simulink model "VVI"  (R2022b)
settings: Solver=FixedStepAuto  StartTime=0.0  StopTime=10.0  FixedStep=1e-3  RelTol=1e-3  EnableMultiTasking=on
undefined symbols (not defined in the file): A0, D1, D10, D12, D2, D5, D9, PTA2, PTB2, PTB9, PTC17, PTC4, PTD0, PTD3
libraries: frdmk64flib x7
settings Model: ExtModeTrigDuration=5  Creator=peter  LastModifiedBy=Dhilan
settings OptimizationCC: EnhancedBackFolding=on  PassReuseOutputArgsAs=Individual arguments  ZeroExternalMemoryAtStartup=off  ZeroInternalMemoryAtStartup=off  MaxStackSize=64  OptimizeBlockOrder=speed  DifferentSizesBufferReuse=on  OptimizationCustomize=off  EfficientTunableParamExpr=on
settings DebuggingCC: ParameterTunabilityLossMsg=error
settings HardwareCC: ProdBitPerPointer=32  ProdBitPerSizeT=32  ProdBitPerPtrDiffT=32  ProdLargestAtomicInteger=Long  ProdLargestAtomicFloat=Double  ProdWordSize=32  ProdHWDeviceType=ARM Compatible->ARM Cortex
settings SFSimCC: MATLABDynamicMemAlloc=off
settings RTWCC: Description=Embedded Coder  SystemTargetFile=ert.tlc  HardwareBoard=NXP FRDM-K64F  TLCOptions="-aInlineSetEventsForThisBaseRateFcn=TLC_FALSE -aSuppressMultiTaskScheduler=TLC_FALSE  -aRateBasedStepFcn=0"  TemplateMakefile=ert_default_tmf  Toolchain=GNU Tools for ARM Embedded Processors  GPUComputeCapability=5.0
settings CodeAppCC: ForceParamTrailComments=on  IgnoreCustomStorageClasses=off  OperatorAnnotations=on  SimulinkDataObjDesc=on  SFDataObjDesc=on  InsertBlockDesc=on
settings ERTTargetCC: ExtModeTransport=4  ExtModeMexFile=sendToCommService

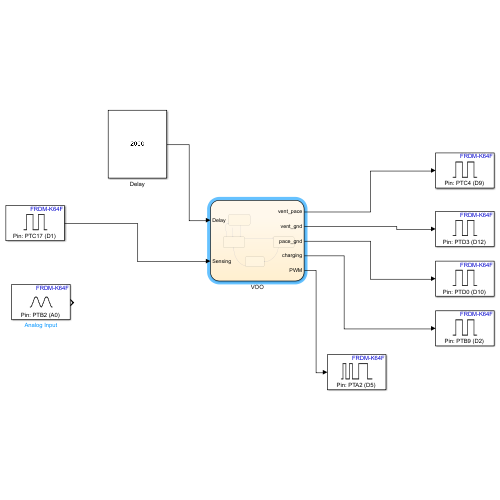
[thumbnail: Simulink's stored preview of the top-level diagram]
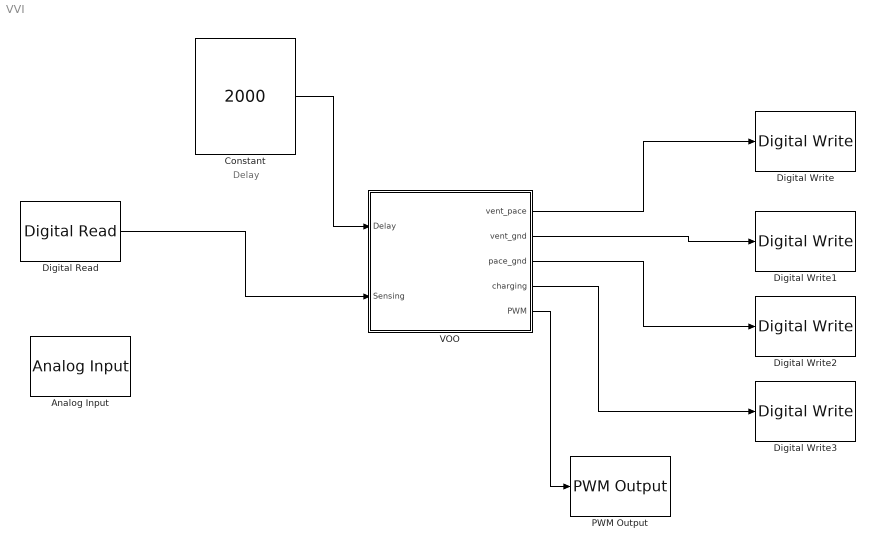
== system VVI ==
  note: Delay
  Analog Input : frdmk64flib/Analog Input  Whichpin=PTB2 (A0)  SampleTime=-1
  Constant : Constant  Value=2000
  Digital Read : frdmk64flib/Digital Read  Whichpin=PTC17 (D1)  SampleTime=-1
  Digital Write : frdmk64flib/Digital Write  Whichpin=PTC4 (D9)
  Digital Write1 : frdmk64flib/Digital Write  Whichpin=PTD3 (D12)
  Digital Write2 : frdmk64flib/Digital Write  Whichpin=PTD0 (D10)
  Digital Write3 : frdmk64flib/Digital Write  Whichpin=PTB9 (D2)
  PWM Output : frdmk64flib/PWM Output  Whichpin=PTA2 (D5)  InitialFrequency=2000  InitialDutyCycle=0
  VOO : Stateflow chart  TreatAsAtomicUnit=on
  wires:
  Constant/1 -> VOO/1(Delay)
  VOO/1(vent_pace) -> Digital Write/1
  VOO/2(vent_gnd) -> Digital Write1/1
  VOO/3(pace_gnd) -> Digital Write2/1
  VOO/4(charging) -> Digital Write3/1
  VOO/5(PWM) -> PWM Output/1
  Digital Read/1 -> VOO/2(Sensing)

== stateflow chart VVI/VOO ==
  state Sensed
  state Charge
    entry:
    PWM = 100;
    charging = true;
  state Pulse
    entry:
    vent_pace = true;
  state Blocking
    entry:
    pace_gnd = true;
    vent_gnd = true;
  Charge -> Sensed [order 1] : [Sensing == 0]
  Sensed -> Charge
  (default) -> Charge
  Charge -> Pulse [order 2] : [after(100,msec)]{charging = false; PWM = 0;}
  Blocking -> Charge : [after(100,msec)]{pace_gnd = false; vent_gnd = false;}
  Pulse -> Blocking : [after(Delay,msec)]{vent_pace = false}
  data: Delay input; vent_pace output; vent_gnd output; pace_gnd output; charging output; PWM output; Sensing input
